simulink library "ddm"  (R2021b)
settings: Solver=VariableStepAuto  StartTime=0.0  StopTime=10.0  RelTol=1e-3
undefined symbols (not defined in the file or in its folder): ADDM_FrTMTqDev_X_Nm, ADDM_RrTMTqDev_X_Nm, ENUM_ADASACCSTA_ERROR, ENUM_ADASACCSTA_OFF, ENUM_ADASACCSTA_STANDBY, ENUM_ALLOWMOV_ALLOWREADY, ENUM_APS, ENUM_BRKSTA_ERROR, ENUM_BRKSTA_OFF, ENUM_BRKSTA_ON, ENUM_BRKSW_INVALID, ENUM_BRKSW_OFF, ENUM_BRKSW_ON, ENUM_CHGPREACTERRSTA_OBCPRE, ENUM_DCDCFAULTSTA_ANYFAULTLV1, ENUM_DCDCFAULTSTA_ANYFAULTLV2, ENUM_DRIVETRAIN_AWD, ENUM_DRIVETRAIN_FWD, ENUM_DRIVETRAIN_RWD, ENUM_EDUDRTSTA_NORMAL, ENUM_EPBSTA_APPLIED, ENUM_EPBSTA_RELEASED, ENUM_GEARACTUALPOSN_INVALID, ENUM_GEARACTUALPOSN_P, ENUM_HVBATTREADYPRE_READY, ENUM_MCUWARN_LV0, ENUM_MCUWARN_LV1, ENUM_MCUWARN_LV2, ENUM_MCUWARN_LV3, ENUM_MCUWARN_NOERROR, ENUM_OBCFAULTSTA_ANYFAULT, ENUM_PAS_R2F2, ENUM_PDFAULT_BATTPDFAIL, ENUM_PDFAULT_DCDCDISABLE, ENUM_PDFAULT_MCUDISABLE, ENUM_PDFAULT_MCUDISCHRG, ENUM_POWERSTA_OFF, ENUM_POWERSTA_ON, ENUM_POWERSTA_READY, ENUM_POWERSTA_STANDBY, ENUM_PRESSINDI_LOW, ENUM_PUFAULT_BATTUPFAIL, ENUM_PUFAULT_DCDCENABLEFAIL, ENUM_PUFAULT_PRECHRGCHKFAIL, ENUM_PUFAULT_SAFETYCHKFAIL, ENUM_PUSTATE_COMPLETED, ENUM_PWRSTASW_OFF, ENUM_PWRSTASW_OFFA, ENUM_PWRSTASW_OFFCHVCHRG, ENUM_PWRSTASW_OFFCLVCHRG, ENUM_PWRSTASW_ON, ENUM_PWRSTASW_ONHVCHRG, ENUM_PWRSTASW_READY, ENUM_PWRSTASW_STANDBY, ENUM_SHIFTCOMMAND_P, ENUM_SHIFTERERRSTA_PBUTTONFAILURE, ENUM_VEHMALFUNLV_2ND, ENUM_VEHMALFUNLV_3RD, ENUM_VEHMALFUNLV_4TH, ENUM_VEHMALFUNLV_NORMAL ... (+459)
libraries: hcu_lib x515, simulink x3
(part 1 of 25)
settings Model: VariantFading=off  Creator=13615  LastModifiedBy=FVT23033
settings SolverCC: AlgebraicLoopSolver=TrustRegion
settings DataIOCC: SaveFormat=Array  SignalLoggingSaveFormat=ModelDataLogs  ReturnWorkspaceOutputs=off
settings OptimizationCC: BlockReduction=off  BooleanDataType=off
settings DebuggingCC: SaveWithParameterizedLinksMsg=none  UnderspecifiedInitializationDetection=Classic  MergeDetectMultiDrivingBlocksExec=none  SignalResolutionControl=TryResolveAllWithWarning  SFMachineParentedDataDiag=warning  ArithmeticOperatorsInVariantConditions=warning
settings HardwareCC: TargetUnknown=on
settings ModelReferenceCC: PropagateSignalLabelsOutOfModel=off
settings SFSimCC: SimUseLocalCustomCode=off  CustomCodeUndefinedFunction=UseInterfaceOnly
settings RTWCC: RTWUseLocalCustomCode=off
settings ConfigComp: CovMetricSettings=dw  CovSaveCumulativeToWorkspaceVar=on  CovSaveSingleToWorkspaceVar=on

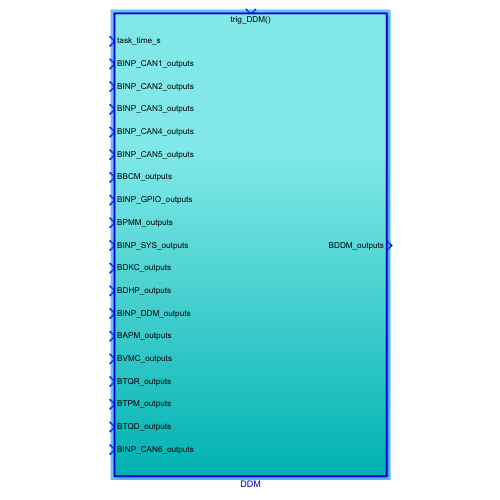
[thumbnail: Simulink's stored preview of the top-level diagram]
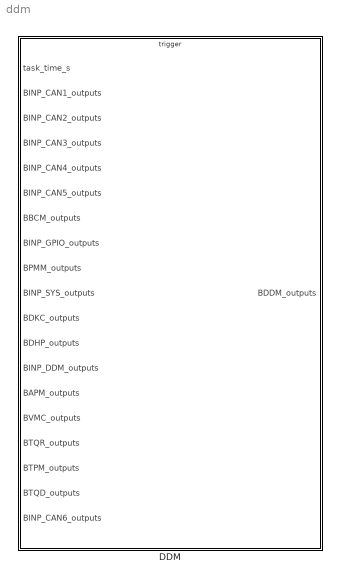
== system ddm ==
  DDM : Subsystem
      settings: RTWSystemCode=Nonreusable function  RTWFcnNameOpts=Use subsystem name  RTWFileNameOpts=Use subsystem name

== system ddm/DDM ==
  task_time_s : Inport
  BINP_CAN1_outputs : Inport  Port=2  OutDataTypeStr=Bus: BINP_CAN1_outputs
  BINP_CAN2_outputs : Inport  Port=3  OutDataTypeStr=Bus: BINP_CAN2_outputs
  BINP_CAN3_outputs : Inport  Port=4  OutDataTypeStr=Bus: BINP_CAN3_outputs
  BINP_CAN4_outputs : Inport  Port=5  OutDataTypeStr=Bus: BINP_CAN4_outputs
  BINP_CAN5_outputs : Inport  Port=6  OutDataTypeStr=Bus: BINP_CAN5_outputs
  BBCM_outputs : Inport  Port=7  OutDataTypeStr=Bus: BBCM_outputs
  BINP_GPIO_outputs : Inport  Port=8  OutDataTypeStr=Bus: BINP_GPIO_outputs
  BPMM_outputs : Inport  Port=9  OutDataTypeStr=Bus: BPMM_outputs
  BINP_SYS_outputs : Inport  Port=10  OutDataTypeStr=Bus: BINP_SYS_outputs
  BDKC_outputs : Inport  Port=11  OutDataTypeStr=Bus: BDKC_outputs
  BDHP_outputs : Inport  Port=12  OutDataTypeStr=Bus: BDHP_outputs
  BINP_DDM_outputs : Inport  Port=13  OutDataTypeStr=Bus: BINP_DDM_outputs
  BAPM_outputs : Inport  Port=14  OutDataTypeStr=Bus: BAPM_outputs
  BVMC_outputs : Inport  Port=15  OutDataTypeStr=Bus: BVMC_outputs
  BTQR_outputs : Inport  Port=16  OutDataTypeStr=Bus: BTQR_outputs
  BTPM_outputs : Inport  Port=17  OutDataTypeStr=Bus: BTPM_outputs
  BTQD_outputs : Inport  Port=18  OutDataTypeStr=Bus: BTQD_outputs
  BINP_CAN6_outputs : Inport  Port=19  OutDataTypeStr=Bus: BINP_CAN6_outputs
  trig_DDM : TriggerPort  TriggerType=function-call  VariantControl=(inherit)
  Bus Creator : BusCreator  Inputs=173  OutDataTypeStr=Bus: BDDM_outputs  NonVirtualBus=on
  Bus Selector : BusSelector  OutputSignals=VINP_CANMsgValidABM1_flg,VINP_BrkPedalPosSta_flg,VINP_BrkPedalPos_pct,VINP_BrkSwSta_flg,VINP_CANMsgValidESC1_flg,VINP_CANMsgValidESC5_flg,VINP_VehSpeed_kph,VINP_ESC1RCErr_flg,VINP_ESC1CSErr_flg,VINP_ESC5RCErr_flg,VINP_ESC5CSErr_flg,VINP_ABM1RCErr_flg,VINP_ABM1CSErr_flg,VINP_EPBSta_enum,VINP_EPBErrSta_enum,VINP_EBDFailed_flg,VINP_HDDFailed_flg,VINP_ABSFailed_flg,VINP_TCSFailed_flg,VINP_ESCFailed_flg,VINP_HBBFailed_flg,VINP_PBAFailed_flg,VINP_HSAFailed_flg,VINP_AVHFailed_flg,VINP_MCPressureV_flg,VINP_BrkSwV_flg,VINP_BrkPedalPosSta_flg,VINP_LongAccelV_flg,VINP_LatAccelV_flg,VINP_YawRateV_flg,VINP_RFPulseCountV_flg,VINP_RRPulseCountV_flg,VINP_LFPulseCountV_flg,VINP_LRPulseCountV_flg,VINP_LRRawWhlSpeedV_flg,VINP_RRRawWhlSpeedV_flg,VINP_LFRawWhlSpeedV_flg,VINP_RFRawWhlSpeedV_flg,VINP_CANMsgValidEPS1_flg,VINP_SASV_flg,VINP_CANMsgValidEPB1_flg,VINP_EPB1RCErr_flg,VINP_EPB1CSErr_flg,VINP_EPS1RCErr_flg,VINP_EPS1CSErr_flg
  Bus Selector1 : BusSelector  OutputSignals=VDHP_EAPCRBAD_flg,VDHP_EAPS1BAD_flg,VDHP_EAPS2BAD_flg,VDHP_EAPS12RangeSta_enum
  Bus Selector10 : BusSelector  OutputSignals=VDKC_DKCAuthSta_enum
  Bus Selector11 : BusSelector  OutputSignals=VVMC_ADASActive_flg,VVMC_APSActive_flg
  Bus Selector12 : BusSelector  OutputSignals=VTQR_FrTMTqReq_Nm,VTQR_RrTMTqReq_Nm
  Bus Selector13 : BusSelector  OutputSignals=VTPM_LFBatWarn_flg,VTPM_RFBatWarn_flg,VTPM_LRBatWarn_flg,VTPM_RRBatWarn_flg,VTPM_LFPressIndi_enum,VTPM_RFPressIndi_enum,VTPM_LRPressIndi_enum,VTPM_RRPressIndi_enum,VTPM_LFWheelTmpIndi_flg,VTPM_RFWheelTmpIndi_flg,VTPM_LRWheelTmpIndi_flg,VTPM_RRWheelTmpIndi_flg,VTPM_LFSensorFail_flg,VTPM_RFSensorFail_flg,VTPM_LRSensorFail_flg,VTPM_RRSensorFail_flg
  Bus Selector14 : BusSelector  OutputSignals=VTQD_ActParkRequest_flg,VTQD_SpdCtrlMode_enum,VTQD_GearActualPosn_enum,VTQD_ExternalTqAllow_flg,VTQD_ExtDoorAllow_flg
  Bus Selector15 : BusSelector  OutputSignals=VINP_CANMsgValidFCM1_flg,VINP_FCM1LifeCount_enum,VINP_FCM1Checksum_enum,VINP_ADASACCSta_enum,VINP_ACCRequiredAccel_mps2
  Bus Selector2 : BusSelector  OutputSignals=VINP_CANMsgValidBMS1_flg,VINP_CANMsgValidBMS6_flg,VINP_CANMsgValidCCU1_flg,VINP_CANMsgValidCCU2_flg,VINP_BMSWarn1_flg,VINP_BMSWarn2_flg,VINP_BMSWarn3_flg,VINP_BMSWarn4_flg,VINP_BMSWarn5_flg,VINP_BMSWarn6_flg,VINP_BMSWarn7_flg,VINP_BMSWarn8_flg,VINP_DCDCFaultSta_enum,VINP_OBCFaultSta_enum,VINP_MCUWarnFNidec_enum,VINP_MCUWarnRNidec_enum,VINP_LVBattDet12V_V,VINP_BMSREADY_flg,VINP_HVBattReady4Pre_enum,VINP_HVBContactorSta_flg,VINP_DCDCReady4Pre_flg,VINP_DCDCEnaSta_flg,VINP_CANMsgValidMCUNF1_flg,VINP_CANMsgValidMCUNR1_flg,VINP_CANMsgValidShifter1_flg,VINP_FrEDUDrtStaNidec_flg,VINP_FrEDURealTMTqNidec_Nm,VINP_RrEDUDrtStaNidec_flg,VINP_RrEDURealTMTqNidec_Nm,VINP_BMS6RCErr_flg,VINP_BMS6CSErr_flg,VINP_BMS1RCErr_flg,VINP_BMS1CSErr_flg,VINP_CCU1RCErr_flg,VINP_CCU1CSErr_flg,VINP_CCU2RCErr_flg,VINP_CCU2CSErr_flg,VINP_MCUNF1RCErr_flg,VINP_MCUNF1CSErr_flg,VINP_MCUNR1RCErr_flg,VINP_MCUNR1CSErr_flg,VINP_Shifter1RCErr_flg,VINP_Shifter1CSErr_flg,VINP_HVBattSOC_pct,VINP_ShifterHandleCmd_enum,VINP_ShifterFailsta_enum,VINP_CANMsgValidBMS5_flg
  Bus Selector3 : BusSelector  OutputSignals=VINP_ClearDTCcmd_flg
  Bus Selector4 : BusSelector  OutputSignals=VBCM_DiagHCrash_flg,VBCM_DiagFLTS_flg,VBCM_DiagFRTS_flg,VBCM_DiagRLTS_flg,VBCM_DiagRRTS_flg
  Bus Selector5 : BusSelector  OutputSignals=VAPM_USSStaFCL_flg,VAPM_USSStaFML_flg,VAPM_USSStaFMR_flg,VAPM_USSStaFCR_flg,VAPM_USSStaRCL_flg,VAPM_USSStaRML_flg,VAPM_USSStaRMR_flg,VAPM_USSStaRCR_flg,VAPM_USSStaFLL_flg,VAPM_USSStaFLR_flg,VAPM_USSStaRLL_flg,VAPM_USSStaRLR_flg,VAPM_SNSRLayout_enum
  Bus Selector6 : BusSelector  OutputSignals=VINP_DrStdAErrSta_flg,VINP_ZoneDrMalfunLevel_enum,VINP_CANMsgValidZONEDRVCU_flg,VINP_CANMsgValidZONEFRVCU_flg,VINP_CANMsgValidDKC1_flg,VINP_CANMsgValidDKC2_flg
  Bus Selector7 : BusSelector  OutputSignals=VINP_BrakeSWGPIO_flg,VINP_BrakeLampSW_flg,VINP_SeatSW_flg,VINP_DrDoorSW_flg,VINP_PsDoorSW_flg,VINP_RLDoorSW_flg,VINP_RRDoorSW_flg,VINP_HoodSW_flg,VINP_TailgateSW_flg,VINP_AccelPedal1Vol_V,VINP_AccelPedal2Vol_V
  Bus Selector8 : BusSelector  OutputSignals=VPMM_PowerSta_enum,VPMM_SysPowerMode_enum,VPMM_PowerUpFault_enum,VPMM_PowerDownFault_enum,VPMM_DrivetrainSelect_enum,VPMM_SafetyChkHLv_flg,VPMM_SafetyChkMLv_flg,VPMM_HVChrgPreActionErrSta_enum,VPMM_MCUReady_flg,VPMM_MCUReady4Pre_flg,VPMM_PowerUpState_enum,VPMM_MCUDCBusMaxVolt_V
  Bus Selector9 : BusSelector  OutputSignals=VINP_AllowMovThd_OTA_enum,VINP_Pedal1Ref5V_V,VINP_Pedal2Ref5V_V,VINP_AuxBattVolmV_mV,VINP_CAN1BusOff_flg,VINP_CAN3BusOff_flg,VINP_CAN4BusOff_flg,VINP_CAN6BusOff_flg
  Constant5 : Constant  Value=ZoneFrMalfunLevel_enum
  DDM : Subsystem
  Ground : Ground
  Terminator : Terminator
  Terminator2 : Terminator
  BDDM_outputs : Outport  OutDataTypeStr=Bus: BDDM_outputs
  wires:
  Bus Selector2/45 -> DDM/91(VINP_ShifterHandleCmd_enum)  "<VINP_ShifterHandleCmd_enum>"
  Bus Selector/14 -> DDM/15(VINP_EPBSta_enum)  "<VINP_EPBSta_enum>"
  Bus Selector14/1 -> DDM/177(VTQD_ActParkRequest_flg)  "<VTQD_ActParkRequest_flg>"
  BTQD_outputs/1 -> Bus Selector14/1
  Bus Selector9/4 -> DDM/121(VINP_AuxBattVolmV_mV)  "<VINP_AuxBattVolmV_mV>"
  Bus Selector2/44 -> DDM/90(VINP_HVBattSOC_pct)  "<VINP_HVBattSOC_pct>"
  Bus Selector9/3 -> DDM/120(VINP_Pedal2Ref5V_V)  "<VINP_Pedal2Ref5V_V>"
  Bus Selector9/2 -> DDM/119(VINP_Pedal1Ref5V_V)  "<VINP_Pedal1Ref5V_V>"
  Bus Selector13/16 -> DDM/176(VTPM_RRSensorFail_flg)  "<VTPM_RRSensorFail_flg>"
  Bus Selector13/15 -> DDM/175(VTPM_LRSensorFail_flg)  "<VTPM_LRSensorFail_flg>"
  Bus Selector13/14 -> DDM/174(VTPM_RFSensorFail_flg)  "<VTPM_RFSensorFail_flg>"
  Bus Selector13/13 -> DDM/173(VTPM_LFSensorFail_flg)  "<VTPM_LFSensorFail_flg>"
  Bus Selector5/13 -> DDM/149(VAPM_SNSRLayout_enum)  "<VAPM_SNSRLayout_enum>"
  Bus Selector13/12 -> DDM/172(VTPM_RRWheelTmpIndi_flg)  "<VTPM_RRWheelTmpIndi_flg>"
  Bus Selector13/11 -> DDM/171(VTPM_LRWheelTmpIndi_flg)  "<VTPM_LRWheelTmpIndi_flg>"
  Bus Selector13/10 -> DDM/170(VTPM_RFWheelTmpIndi_flg)  "<VTPM_RFWheelTmpIndi_flg>"
  Bus Selector13/9 -> DDM/169(VTPM_LFWheelTmpIndi_flg)  "<VTPM_LFWheelTmpIndi_flg>"
  Bus Selector13/8 -> DDM/168(VTPM_RRPressIndi_enum)  "<VTPM_RRPressIndi_enum>"
  Bus Selector13/7 -> DDM/167(VTPM_LRPressIndi_enum)  "<VTPM_LRPressIndi_enum>"
  Bus Selector13/6 -> DDM/166(VTPM_RFPressIndi_enum)  "<VTPM_RFPressIndi_enum>"
  Bus Selector13/5 -> DDM/165(VTPM_LFPressIndi_enum)  "<VTPM_LFPressIndi_enum>"
  Bus Selector/13 -> DDM/14(VDDM_C1ABM1CSChk_flg)  "<VINP_ABM1CSErr_flg>"
  Bus Selector/12 -> DDM/13(VDDM_C1ABM1RCChk_flg)  "<VINP_ABM1RCErr_flg>"
  Bus Selector/11 -> DDM/12(VDDM_ESC5CSErr_flg)  "<VINP_ESC5CSErr_flg>"
  Bus Selector/10 -> DDM/11(VDDM_ESC5RCErr_flg)  "<VINP_ESC5RCErr_flg>"
  Bus Selector/9 -> DDM/10(VDDM_ESC1CSErr_flg)  "<VINP_ESC1CSErr_flg>"
  Bus Selector/8 -> DDM/9(VDDM_ESC1RCErr_flg)  "<VINP_ESC1RCErr_flg>"
  Bus Selector2/43 -> DDM/89(VDDM_Shifter1CSErr_flg)  "<VINP_Shifter1CSErr_flg>"
  Bus Selector2/42 -> DDM/88(VDDM_Shifter1RCErr_flg)  "<VINP_Shifter1RCErr_flg>"
  Bus Selector2/41 -> DDM/87(VDDM_MCUNR1CSErr_flg)  "<VINP_MCUNR1CSErr_flg>"
  Bus Selector2/40 -> DDM/86(VDDM_MCUNR1RCErr_flg)  "<VINP_MCUNR1RCErr_flg>"
  Bus Selector2/39 -> DDM/85(VDDM_MCUNF1CSErr_flg)  "<VINP_MCUNF1CSErr_flg>"
  Bus Selector2/38 -> DDM/84(VDDM_MCUNF1RCErr_flg)  "<VINP_MCUNF1RCErr_flg>"
  Bus Selector2/37 -> DDM/83(VDDM_C3CCU2CSChk_flg)  "<VINP_CCU2CSErr_flg>"
  Bus Selector2/36 -> DDM/82(VDDM_C3CCU2RCChk_flg)  "<VINP_CCU2RCErr_flg>"
  Bus Selector2/35 -> DDM/81(VDDM_C3CCU1CSChk_flg)  "<VINP_CCU1CSErr_flg>"
  Bus Selector2/34 -> DDM/80(VDDM_C3CCU1RCChk_flg)  "<VINP_CCU1RCErr_flg>"
  Bus Selector2/33 -> DDM/79(VDDM_C3BMS1CSChk_flg)  "<VINP_BMS1CSErr_flg>"
  Bus Selector2/32 -> DDM/78(VDDM_C3BMS1RCChk_flg)  "<VINP_BMS1RCErr_flg>"
  Bus Selector2/31 -> DDM/77(VDDM_C3BMS6CSChk_flg)  "<VINP_BMS6CSErr_flg>"
  Bus Selector2/30 -> DDM/76(VDDM_C3BMS6RCChk_flg)  "<VINP_BMS6RCErr_flg>"
  Bus Selector13/4 -> DDM/164(VTPM_RRBatwarn_flg)  "<VTPM_RRBatWarn_flg>"
  Bus Selector13/3 -> DDM/163(VTPM_LRBatwarn_flg)  "<VTPM_LRBatWarn_flg>"
  Bus Selector13/2 -> DDM/162(VTPM_RFBatwarn_flg)  "<VTPM_RFBatWarn_flg>"
  Bus Selector13/1 -> DDM/161(VTPM_LFBatwarn_flg)  "<VTPM_LFBatWarn_flg>"
  BTPM_outputs/1 -> Bus Selector13/1
  Bus Selector12/2 -> DDM/160(VTQR_RrTMTqReq_Nm)  "<VTQR_RrTMTqReq_Nm>"
  Bus Selector12/1 -> DDM/159(VTQR_FrTMTqReq_Nm)  "<VTQR_FrTMTqReq_Nm>"
  BTQR_outputs/1 -> Bus Selector12/1
  Bus Selector2/29 -> DDM/75(VINP_RrEDURealTMTqNidec_Nm)  "<VINP_RrEDURealTMTqNidec_Nm>"
  Bus Selector2/28 -> DDM/74(VINP_RrEDUDrtStaNidec_flg)  "<VINP_RrEDUDrtStaNidec_flg>"
  Bus Selector2/27 -> DDM/73(VINP_FrEDURealTMTqNidec_Nm)  "<VINP_FrEDURealTMTqNidec_Nm>"
  Bus Selector2/26 -> DDM/72(VINP_FrEDUDrtStaNidec_flg)  "<VINP_FrEDUDrtStaNidec_flg>"
  Bus Selector/7 -> DDM/8(VINP_VehSpeed_kph)  "<VINP_VehSpeed_kph>"
  Bus Selector11/1 -> DDM/157(VVMC_ADASActive_flg)  "<VVMC_ADASActive_flg>"
  BVMC_outputs/1 -> Bus Selector11/1
  Bus Selector5/12 -> DDM/148(VAPM_USSStaRLR_flg)  "<VAPM_USSStaRLR_flg>"
  Bus Selector5/11 -> DDM/147(VAPM_USSStaRLL_flg)  "<VAPM_USSStaRLL_flg>"
  Bus Selector5/10 -> DDM/146(VAPM_USSStaFLR_flg)  "<VAPM_USSStaFLR_flg>"
  Bus Selector5/9 -> DDM/145(VAPM_USSStaFLL_flg)  "<VAPM_USSStaFLL_flg>"
  Bus Selector5/8 -> DDM/144(VAPM_USSStaRCR_flg)  "<VAPM_USSStaRCR_flg>"
  Bus Selector5/7 -> DDM/143(VAPM_USSStaRMR_flg)  "<VAPM_USSStaRMR_flg>"
  Bus Selector5/6 -> DDM/142(VAPM_USSStaRML_flg)  "<VAPM_USSStaRML_flg>"
  Bus Selector5/5 -> DDM/141(VAPM_USSStaRCL_flg)  "<VAPM_USSStaRCL_flg>"
  Bus Selector5/4 -> DDM/140(VAPM_USSStaFCR_flg)  "<VAPM_USSStaFCR_flg>"
  Bus Selector5/3 -> DDM/139(VAPM_USSStaFMR_flg)  "<VAPM_USSStaFMR_flg>"
  Bus Selector5/1 -> DDM/137(VAPM_USSStaFCL_flg)  "<VAPM_USSStaFCL_flg>"
  Bus Selector5/2 -> DDM/138(VAPM_USSStaFML_flg)  "<VAPM_USSStaFML_flg>"
  BAPM_outputs/1 -> Bus Selector5/1
  Bus Selector8/11 -> DDM/104(VPMM_PowerUpState_enum)  "<VPMM_PowerUpState_enum>"
  Bus Selector3/1 -> DDM/127(DTC_clear_request)  "<VINP_ClearDTCcmd_flg>"
  Bus Selector2/25 -> DDM/71(VINP_CANMsgValidShifter1_flg)  "<VINP_CANMsgValidShifter1_flg>"
  Bus Selector2/24 -> DDM/70(VINP_CANMsgValidMCUNR1_flg)  "<VINP_CANMsgValidMCUNR1_flg>"
  Bus Selector2/23 -> DDM/69(VINP_CANMsgValidMCUNF1_flg)  "<VINP_CANMsgValidMCUNF1_flg>"
  Bus Selector/6 -> DDM/7(VINP_CANMsgValidESC5_flg)  "<VINP_CANMsgValidESC5_flg>"
  Bus Selector/5 -> DDM/6(VINP_CANMsgValidESC1_flg)  "<VINP_CANMsgValidESC1_flg>"
  Bus Selector4/5 -> DDM/136(VBCM_DiagRRTS_flg)  "<VBCM_DiagRRTS_flg>"
  Bus Selector4/4 -> DDM/135(VBCM_DiagRLTS_flg)  "<VBCM_DiagRLTS_flg>"
  Bus Selector4/3 -> DDM/134(VBCM_DiagFRTS_flg)  "<VBCM_DiagFRTS_flg>"
  Bus Selector4/2 -> DDM/133(VBCM_DiagFLTS_flg)  "<VBCM_DiagFLTS_flg>"
  Bus Selector4/1 -> DDM/132(VBCM_DiagHCrash_flg)  "<VBCM_DiagHCrash_flg>"
  BINP_DDM_outputs/1 -> Bus Selector3/1
  Bus Selector8/10 -> DDM/103(VPMM_MCUReady4Pre_flg)  "<VPMM_MCUReady4Pre_flg>"
  Bus Selector8/9 -> DDM/102(VPMM_MCUReady_flg)  "<VPMM_MCUReady_flg>"
  Bus Selector8/8 -> DDM/101(VPMM_HVChrgPreActionErrSta_enum)  "<VPMM_HVChrgPreActionErrSta_enum>"
  Bus Selector8/7 -> DDM/100(VPMM_SafetyChkMLv_flg)  "<VPMM_SafetyChkMLv_flg>"
  Bus Selector8/6 -> DDM/99(VPMM_SafetyChkHLv_flg)  "<VPMM_SafetyChkHLv_flg>"
  Bus Selector1/1 -> DDM/128(VDHP_EAPCRBAD_flg)  "<VDHP_EAPCRBAD_flg>"
  BDHP_outputs/1 -> Bus Selector1/1
  Bus Selector7/11 -> DDM/116(VINP_AccelPedal2Vol_V)  "<VINP_AccelPedal2Vol_V>"
  Bus Selector7/10 -> DDM/115(VINP_AccelPedal1Vol_V)  "<VINP_AccelPedal1Vol_V>"
  DDM/39(VDDM_LVSupHiDTC_raw32) -> Bus Creator/39
  DDM/38(VDDM_LVSupLoDTC_raw32) -> Bus Creator/38
  DDM/37(VDDM_IniLVLoDTC_raw32) -> Bus Creator/37
  DDM/36(VDDM_OBC4PreDTC_raw32) -> Bus Creator/36
  DDM/35(VDDM_MCUActDTC_raw32) -> Bus Creator/35
  DDM/34(VDDM_HVRlyOpDTC_raw32) -> Bus Creator/34
  DDM/33(VDDM_DCDCDisDTC_raw32) -> Bus Creator/33
  DDM/32(VDDM_MCUDisDTC_raw32) -> Bus Creator/32
  DDM/31(VDDM_MidLvSaChkDTC_raw32) -> Bus Creator/31
  DDM/30(VDDM_HiLvSaChkDTC_raw32) -> Bus Creator/30
  DDM/29(VDDM_DCDCEnaDTC_raw32) -> Bus Creator/29
  DDM/28(VDDM_BMSRdyDTC_raw32) -> Bus Creator/28
  DDM/27(VDDM_HVRlyCloDTC_raw32) -> Bus Creator/27
  DDM/26(VDDM_DCDC4PreDTC_raw32) -> Bus Creator/26
  DDM/25(VDDM_MCU4PreDTC_raw32) -> Bus Creator/25
  DDM/24(VDDM_HVB4PreDTC_raw32) -> Bus Creator/24
  DDM/23(VDDM_ONtoRdyDTC_raw32) -> Bus Creator/23
  DDM/22(VDDM_KeyAuthDTC_raw32) -> Bus Creator/22
  DDM/21(VDDM_BrkSWNoBacDTC_raw32) -> Bus Creator/21
  DDM/20(VDDM_BrkSWErrDTC_raw32) -> Bus Creator/20
  DDM/19(VDDM_Lv4ErrDTC_raw32) -> Bus Creator/19
  DDM/18(VDDM_Lv3ErrDTC_raw32) -> Bus Creator/18
  DDM/17(VDDM_Lv2ErrDTC_raw32) -> Bus Creator/17
  DDM/1(VDDM_C3BMS6RCDTC_raw32) -> Bus Creator/1
  DDM/16(VDDM_Lv1ErrDTC_raw32) -> Bus Creator/16
  DDM/2(VDDM_C3BMS6CSDTC_raw32) -> Bus Creator/2
  DDM/15(VDDM_C1ABM1LCDTC_raw32) -> Bus Creator/15
  DDM/3(VDDM_C3BMS6LCDTC_raw32) -> Bus Creator/3
  DDM/14(VDDM_C1ABM1CSDTC_raw32) -> Bus Creator/14
  DDM/4(VDDM_C3BMS1RCDTC_raw32) -> Bus Creator/4
  DDM/13(VDDM_C1ABM1RCDTC_raw32) -> Bus Creator/13
  DDM/5(VDDM_C3BMS1CSDTC_raw32) -> Bus Creator/5
  DDM/12(VDDM_C3CCU2LCDTC_raw32) -> Bus Creator/12
  DDM/6(VDDM_C3BMS1LCDTC_raw32) -> Bus Creator/6
  DDM/11(VDDM_C3CCU2CSDTC_raw32) -> Bus Creator/11
  DDM/7(VDDM_C3CCU1RCDTC_raw32) -> Bus Creator/7
  DDM/10(VDDM_C3CCU2RCDTC_raw32) -> Bus Creator/10
  DDM/8(VDDM_C3CCU1CSDTC_raw32) -> Bus Creator/8
  DDM/9(VDDM_C3CCU1LCDTC_raw32) -> Bus Creator/9
  BBCM_outputs/1 -> Bus Selector4/1
  BINP_CAN5_outputs/1 -> Terminator2/1
  BINP_CAN4_outputs/1 -> Bus Selector6/1
  BINP_CAN2_outputs/1 -> Terminator/1
  Bus Selector7/3 -> DDM/108(VINP_DrStSW)  "<VINP_SeatSW_flg>"
  Bus Selector7/4 -> DDM/109(VINP_FLAJARSW)  "<VINP_DrDoorSW_flg>"
  Bus Selector7/5 -> DDM/110(VINP_FRAJARSW)  "<VINP_PsDoorSW_flg>"
  Bus Selector7/6 -> DDM/111(VINP_RLAJARSW)  "<VINP_RLDoorSW_flg>"
  Bus Selector7/7 -> DDM/112(VINP_RRAJARSW)  "<VINP_RRDoorSW_flg>"
  Bus Selector7/8 -> DDM/113(VINP_HoodSW)  "<VINP_HoodSW_flg>"
  Bus Selector7/9 -> DDM/114(VINP_TailgaSW)  "<VINP_TailgateSW_flg>"
  Bus Selector/4 -> DDM/5(VINP_BrkSWSta_flg)  "<VINP_BrkSwSta_flg>"
  Bus Selector2/22 -> DDM/68(VINP_DCDCEnabled_flg)  "<VINP_DCDCEnaSta_flg>"
  Bus Selector10/1 -> DDM/117(VDKC_DKCAuthSta_enum)  "<VDKC_DKCAuthSta_enum>"
  BDKC_outputs/1 -> Bus Selector10/1
  Bus Selector9/1 -> DDM/118(VINP_AllowMovThd_OTA_enum)  "<VINP_AllowMovThd_OTA_enum>"
  BINP_SYS_outputs/1 -> Bus Selector9/1
  Bus Selector7/2 -> DDM/107(VINP_BrakeLampSW_flg)  "<VINP_BrakeLampSW_flg>"
  Bus Selector7/1 -> DDM/106(VINP_BrakeSWGPIO_flg)  "<VINP_BrakeSWGPIO_flg>"
  Bus Selector8/5 -> DDM/98(VPMM_DrivetrainSelect_enum)  "<VPMM_DrivetrainSelect_enum>"
  Bus Selector8/4 -> DDM/97(VPMM_PowerDownFault_enum)  "<VPMM_PowerDownFault_enum>"
  Bus Selector8/3 -> DDM/96(VPMM_PowerUpFault_enum)  "<VPMM_PowerUpFault_enum>"
  Bus Selector8/2 -> DDM/95(VPMM_PwrStaSW_enum)  "<VPMM_SysPowerMode_enum>"
  Bus Selector8/1 -> DDM/94(VPMM_PowerSta_enum)  "<VPMM_PowerSta_enum>"
  Bus Selector2/21 -> DDM/67(VINP_DCDCReady4Pre_flg)  "<VINP_DCDCReady4Pre_flg>"
  Bus Selector2/20 -> DDM/66(VINP_HVBContactorSta_flg)  "<VINP_HVBContactorSta_flg>"
  Bus Selector2/19 -> DDM/65(VINP_HVBattReady4Pre_enum)  "<VINP_HVBattReady4Pre_enum>"
  Bus Selector2/18 -> DDM/64(VINP_BMSREADY_flg)  "<VINP_BMSREADY_flg>"
  Bus Selector2/17 -> DDM/63(VINP_LVBattDet12V_V)  "<VINP_LVBattDet12V_V>"
  Bus Selector2/16 -> DDM/62(VINP_MCUWarnRNidec_enum)  "<VINP_MCUWarnRNidec_enum>"
  Bus Selector2/15 -> DDM/61(VINP_MCUWarnFNidec_enum)  "<VINP_MCUWarnFNidec_enum>"
  Bus Selector2/14 -> DDM/60(VINP_OBCFaultSta_enum)  "<VINP_OBCFaultSta_enum>"
  Bus Selector2/13 -> DDM/59(VINP_DCDCFaultSta_enum)  "<VINP_DCDCFaultSta_enum>"
  Bus Selector2/12 -> DDM/58(VINP_BMSWarn8_flg)  "<VINP_BMSWarn8_flg>"
  Bus Selector2/11 -> DDM/57(VINP_BMSWarn7_flg)  "<VINP_BMSWarn7_flg>"
  Bus Selector2/10 -> DDM/56(VINP_BMSWarn6_flg)  "<VINP_BMSWarn6_flg>"
  Bus Selector2/9 -> DDM/55(VINP_BMSWarn5_flg)  "<VINP_BMSWarn5_flg>"
  Bus Selector2/8 -> DDM/54(VINP_BMSWarn4_flg)  "<VINP_BMSWarn4_flg>"
  Bus Selector2/7 -> DDM/53(VINP_BMSWarn3_flg)  "<VINP_BMSWarn3_flg>"
  Bus Selector2/6 -> DDM/52(VINP_BMSWarn2_flg)  "<VINP_BMSWarn2_flg>"
  Bus Selector2/1 -> DDM/47(VINP_CANMsgValidBMS1_flg)  "<VINP_CANMsgValidBMS1_flg>"
  Bus Selector2/5 -> DDM/51(VINP_BMSWarn1_flg)  "<VINP_BMSWarn1_flg>"
  Bus Selector2/2 -> DDM/48(VINP_CANMsgValidBMS6_flg)  "<VINP_CANMsgValidBMS6_flg>"
  Bus Selector2/4 -> DDM/50(VINP_CANMsgValidCCU2_flg)  "<VINP_CANMsgValidCCU2_flg>"
  Bus Selector2/3 -> DDM/49(VINP_CANMsgValidCCU1_flg)  "<VINP_CANMsgValidCCU1_flg>"
  Bus Selector/3 -> DDM/4(VINP_BrkPedalPos_pct)  "<VINP_BrkPedalPos_pct>"
  Bus Selector/2 -> DDM/3(VINP_BrkPedalPosSta_enum)  "<VINP_BrkPedalPosSta_flg>"
  Bus Selector/1 -> DDM/2(VINP_CANMsgValidABM1_flg)  "<VINP_CANMsgValidABM1_flg>"
  BPMM_outputs/1 -> Bus Selector8/1
  Bus Creator/1 -> BDDM_outputs/1  "BDDM_outputs"
  task_time_s/1 -> DDM/1(task_time_s)
  BINP_GPIO_outputs/1 -> Bus Selector7/1
  BINP_CAN3_outputs/1 -> Bus Selector2/1
  BINP_CAN1_outputs/1 -> Bus Selector/1
  Bus Selector6/1 -> DDM/150(VINP_DrStdAErrSta_enum)  "<VINP_DrStdAErrSta_flg>"
  Bus Selector6/2 -> DDM/151(VINP_ZoneDrMalfunLevel_enum)  "<VINP_ZoneDrMalfunLevel_enum>"
  Bus Selector15/1 -> DDM/182(VINP_CANMsgValidFCM1_flg)  "<VINP_CANMsgValidFCM1_flg>"
  Bus Selector14/2 -> DDM/178(VINP_ZoneSpdCtrlMode_enum)  "<VTQD_SpdCtrlMode_enum>"
  Bus Selector2/46 -> DDM/92(VINP_ShifterFailsta_enum)  "<VINP_ShifterFailsta_enum>"
  Constant5/1 -> DDM/156(ZoneFrMalfunLevel_enum)
  Bus Selector8/12 -> DDM/105(VPMM_MCUDCBusMaxVolt_V)  "<VPMM_MCUDCBusMaxVolt_V>"
  Bus Selector14/3 -> DDM/179(VTQD_GearActualPosn_enum)  "<VTQD_GearActualPosn_enum>"
  Bus Selector/15 -> DDM/16(VINP_EPBErrSta_enum)  "<VINP_EPBErrSta_enum>"
  Bus Selector/41 -> DDM/42(VINP_CANMsgValidEPB1_flg)  "<VINP_CANMsgValidEPB1_flg>"
  Bus Selector1/2 -> DDM/129(VDHP_EAPS1BAD_flg)  "<VDHP_EAPS1BAD_flg>"
  Bus Selector1/3 -> DDM/130(VDHP_EAPS2BAD_flg)  "<VDHP_EAPS2BAD_flg>"
  BINP_CAN6_outputs/1 -> Bus Selector15/1
  Bus Selector15/2 -> DDM/183(VDDM_FCM1RCErr_flg)  "<VINP_FCM1LifeCount_enum>"
  Bus Selector15/3 -> DDM/184(VDDM_FCM1CSErr_flg)  "<VINP_FCM1Checksum_enum>"
  Bus Selector15/4 -> DDM/185(VINP_ADASACCSta_enum)  "<VINP_ADASACCSta_enum>"
  Bus Selector15/5 -> DDM/186(VINP_ACCRequireAccel_mps2)  "<VINP_ACCRequiredAccel_mps2>"
  Bus Selector14/4 -> DDM/180(VTQD_ExternalTqAllow_flg)  "<VTQD_ExternalTqAllow_flg>"
  Bus Selector14/5 -> DDM/181(VTQD_ExtDoorAllow_flg)  "<VTQD_ExtDoorAllow_flg>"
  Bus Selector/38 -> DDM/39(VINP_RFRawWhlSpeedV_flg)  "<VINP_RFRawWhlSpeedV_flg>"
  Bus Selector/37 -> DDM/38(VINP_LFRawWhlSpeedV_flg)  "<VINP_LFRawWhlSpeedV_flg>"
  Bus Selector/36 -> DDM/37(VINP_RRRawWhlSpeedV_flg)  "<VINP_RRRawWhlSpeedV_flg>"
  Bus Selector/35 -> DDM/36(VINP_LRRawWhlSpeedV_flg)  "<VINP_LRRawWhlSpeedV_flg>"
  Bus Selector/34 -> DDM/35(VINP_LRPulseCountV_flg)  "<VINP_LRPulseCountV_flg>"
  Bus Selector/33 -> DDM/34(VINP_LFPulseCountV_flg)  "<VINP_LFPulseCountV_flg>"
  Bus Selector/32 -> DDM/33(VINP_RRPulseCountV_flg)  "<VINP_RRPulseCountV_flg>"
  Bus Selector/31 -> DDM/32(VINP_RFPulseCountV_flg)  "<VINP_RFPulseCountV_flg>"
  Bus Selector/30 -> DDM/31(VINP_YawRateV_flg)  "<VINP_YawRateV_flg>"
  Bus Selector/29 -> DDM/30(VINP_LatAccelV_flg)  "<VINP_LatAccelV_flg>"
  Bus Selector/28 -> DDM/29(VINP_LongAccelV_flg)  "<VINP_LongAccelV_flg>"
  Bus Selector/27 -> DDM/28(VINP_BrkPedalPosSta_flg)  "<VINP_BrkPedalPosSta_flg>"
  Bus Selector/26 -> DDM/27(VINP_BrkSwV_flg)  "<VINP_BrkSwV_flg>"
  Bus Selector/25 -> DDM/26(VINP_MCPressureV_flg)  "<VINP_MCPressureV_flg>"
  Bus Selector/24 -> DDM/25(VINP_AVHFailed_flg)  "<VINP_AVHFailed_flg>"
  Bus Selector/23 -> DDM/24(VINP_HSAFailed_flg)  "<VINP_HSAFailed_flg>"
  Bus Selector/22 -> DDM/23(VINP_PBAFailed_flg)  "<VINP_PBAFailed_flg>"
  Bus Selector/21 -> DDM/22(VINP_HBBFailed_flg)  "<VINP_HBBFailed_flg>"
  Bus Selector/20 -> DDM/21(VINP_ESCFailed_flg)  "<VINP_ESCFailed_flg>"
  Bus Selector/19 -> DDM/20(VINP_TCSFailed_flg)  "<VINP_TCSFailed_flg>"
  Bus Selector/18 -> DDM/19(VINP_ABSFailed_flg)  "<VINP_ABSFailed_flg>"
  Bus Selector/17 -> DDM/18(VINP_HDDFailed_flg)  "<VINP_HDDFailed_flg>"
  Bus Selector/16 -> DDM/17(VINP_EBDFailed_flg)  "<VINP_EBDFailed_flg>"
  Bus Selector/39 -> DDM/40(VINP_CANMsgValidEPS1_flg)  "<VINP_CANMsgValidEPS1_flg>"
  Bus Selector/40 -> DDM/41(VINP_SASV_flg)  "<VINP_SASV_flg>"
  DDM/40(VDDM_LVInErrDTC_raw32) -> Bus Creator/40
  DDM/41(VDDM_DrStSWDTC_raw32) -> Bus Creator/41
  DDM/42(VDDM_FLDoorSWDTC_raw32) -> Bus Creator/42
  DDM/43(VDDM_RLDoorSWDTC_raw32) -> Bus Creator/43
  DDM/44(VDDM_FRDoorSWDTC_raw32) -> Bus Creator/44
  DDM/45(VDDM_RRDoorSWDTC_raw32) -> Bus Creator/45
  DDM/46(VDDM_HoodSWDTC_raw32) -> Bus Creator/46
  DDM/47(VDDM_TailgaSWDTC_raw32) -> Bus Creator/47
  DDM/48(VDDM_EDriveSysErrVCUErr_flg) -> Bus Creator/48
  DDM/49(VDDM_VehMalfunLevel_enum) -> Bus Creator/49
  DDM/50(VDDM_APS1SigOoRDTC_raw32) -> Bus Creator/50
  DDM/51(VDDM_APS2SigOoRDTC_raw32) -> Bus Creator/51
  DDM/52(VDDM_APSCorrErrDTC_raw32) -> Bus Creator/52
  DDM/53(VDDM_MCUF1NoComDTC_raw32) -> Bus Creator/53
  DDM/54(VDDM_MCUR1NoComDTC_raw32) -> Bus Creator/54
  DDM/55(VDDM_Shifter1NoComDTC_raw32) -> Bus Creator/55
  DDM/56(VDDM_ESC7NoComDTC_raw32) -> Bus Creator/56
  DDM/57(VDDM_ESC1NoComDTC_raw32) -> Bus Creator/57
  DDM/58(VDDM_ESC5NoComDTC_raw32) -> Bus Creator/58
  DDM/59(VDDM_EnterNewOperCyc_flg) -> Bus Creator/59
  DDM/60(VDDM_DiagHCrashDTC_raw32) -> Bus Creator/60
  DDM/61(VDDM_DiagFLTSDTC_raw32) -> Bus Creator/61
  DDM/62(VDDM_DiagFRTSDTC_raw32) -> Bus Creator/62
  DDM/63(VDDM_DiagRLTSDTC_raw32) -> Bus Creator/63
  DDM/64(VDDM_DiagRRTSDTC_raw32) -> Bus Creator/64
  DDM/65(VDDM_FCLUSSDTC_raw32) -> Bus Creator/65
  DDM/66(VDDM_FMLUSSDTC_raw32) -> Bus Creator/66
  DDM/67(VDDM_FMRUSSDTC_raw32) -> Bus Creator/67
  DDM/68(VDDM_FCRUSSDTC_raw32) -> Bus Creator/68
  DDM/69(VDDM_RCLUSSDTC_raw32) -> Bus Creator/69
  DDM/70(VDDM_RMLUSSDTC_raw32) -> Bus Creator/70
  DDM/71(VDDM_RMRUSSDTC_raw32) -> Bus Creator/71
  DDM/72(VDDM_RCRUSSDTC_raw32) -> Bus Creator/72
  DDM/73(VDDM_FLLUSSDTC_raw32) -> Bus Creator/73
  DDM/74(VDDM_FLRUSSDTC_raw32) -> Bus Creator/74
  DDM/75(VDDM_RLLUSSDTC_raw32) -> Bus Creator/75
  DDM/76(VDDM_RLRUSSDTC_raw32) -> Bus Creator/76
  DDM/77(VDDM_FCM2NoComDTC_raw32) -> Bus Creator/77
  DDM/78(VDDM_FCM2RCErrDTC_raw32) -> Bus Creator/78
  DDM/79(VDDM_FCM2CSErrDTC_raw32) -> Bus Creator/79
  DDM/81(VDDM_FCM3RCErrDTC_raw32) -> Bus Creator/81
  DDM/80(VDDM_FCM3NoComDTC_raw32) -> Bus Creator/80
  DDM/82(VDDM_FCM3CSErrDTC_raw32) -> Bus Creator/82
  DDM/83(VDDM_FCM4NoComDTC_raw32) -> Bus Creator/83
  DDM/84(VDDM_FCM4CSErrDTC_raw32) -> Bus Creator/84
  DDM/85(VDDM_FCM5NoComDTC_raw32) -> Bus Creator/85
  DDM/86(VDDM_FCM5CSErrDTC_raw32) -> Bus Creator/86
  DDM/87(VDDM_ZoneSCPNoComDTC_raw32) -> Bus Creator/87
  DDM/88(VDDM_BMSSigErrDetDTC_raw32) -> Bus Creator/88
  DDM/89(VDDM_FCMACCSigErrDetDTC_raw32) -> Bus Creator/89
  DDM/90(VDDM_FrMCUSigErrDetDTC_raw32) -> Bus Creator/90
  DDM/91(VDDM_RrMCUSigErrDetDTC_raw32) -> Bus Creator/91
  DDM/92(VDDM_CCUSigErrDetDTC_raw32) -> Bus Creator/92
  DDM/93(VDDM_ACCAccelCmdErrDetDTC_raw32) -> Bus Creator/93
  DDM/94(VDDM_ACCMalfuncDetDTC_raw32) -> Bus Creator/94
  DDM/95(VDDM_CCMalfuncDetDTC_raw32) -> Bus Creator/95
  DDM/96(VDDM_MSAMalfuncDetDTC_raw32) -> Bus Creator/96
  DDM/97(VDDM_ISAMalfuncDetDTC_raw32) -> Bus Creator/97
  DDM/98(VDDM_MCUF1RCErrDTC_raw32) -> Bus Creator/98
  DDM/99(VDDM_MCUR1RCErrDTC_raw32) -> Bus Creator/99
  DDM/100(VDDM_MCUF1CSErrDTC_raw32) -> Bus Creator/100
  DDM/101(VDDM_MCUR1CSErrDTC_raw32) -> Bus Creator/101
  DDM/102(VDDM_Shifter1RCErrDTC_raw32) -> Bus Creator/102
  DDM/103(VDDM_Shifter1CSErrDTC_raw32) -> Bus Creator/103
  DDM/104(VDDM_ESC7RCErrDTC_raw32) -> Bus Creator/104
  DDM/105(VDDM_ESC7CSErrDTC_raw32) -> Bus Creator/105
  DDM/106(VDDM_ESC1RCErrDTC_raw32) -> Bus Creator/106
  DDM/107(VDDM_ESC1CSErrDTC_raw32) -> Bus Creator/107
  DDM/108(VDDM_ESC5RCErrDTC_raw32) -> Bus Creator/108
  DDM/109(VDDM_ESC5C  SErrDTC_raw32) -> Bus Creator/109
  DDM/110(VDDM_FrMCUTqErrDTC_raw32) -> Bus Creator/110
  DDM/111(VDDM_RrMCUTqErrDTC_raw32) -> Bus Creator/111
  DDM/112(VDDM_LFBatwarnDTC_raw32) -> Bus Creator/112
  DDM/113(VDDM_RFBatwarnDTC_raw32) -> Bus Creator/113
  DDM/114(VDDM_LRBatwarnDTC_raw32) -> Bus Creator/114
  DDM/115(VDDM_RRBatwarnDTC_raw32) -> Bus Creator/115
  DDM/116(VDDM_LFPressIndiDTC_raw32) -> Bus Creator/116
  DDM/117(VDDM_RFPressIndiDTC_raw32) -> Bus Creator/117
  DDM/118(VDDM_LRPressIndiDTC_raw32) -> Bus Creator/118
  DDM/119(VDDM_RRPressIndiDTC_raw32) -> Bus Creator/119
  DDM/120(VDDM_LFWheelTmpHighDTC_raw32) -> Bus Creator/120
  DDM/121(VDDM_RFWheelTmpHighDTC_raw32) -> Bus Creator/121
  DDM/122(VDDM_LRWheelTmpHighDTC_raw32) -> Bus Creator/122
  DDM/123(VDDM_RRWheelTmpHighDTC_raw32) -> Bus Creator/123
  DDM/124(VDDM_LFSensorFailDTC_raw32) -> Bus Creator/124
  DDM/125(VDDM_RFSensorFailDTC_raw32) -> Bus Creator/125
  DDM/126(VDDM_LRSensorFailDTC_raw32) -> Bus Creator/126
  DDM/127(VDDM_RRSensorFailDTC_raw32) -> Bus Creator/127
  DDM/128(VDDM_C1EPAS2LCDTC_raw32) -> Bus Creator/128
  DDM/129(VDDM_5vAPS1PwrErrDTC_raw32) -> Bus Creator/129
  DDM/151(VDDM_EPSSigErrDTC_raw32) -> Bus Creator/151
  DDM/150(VDDM_EPS1CSErrDTC_raw32) -> Bus Creator/150
  DDM/149(VDDM_EPS1RCErrDTC_raw32) -> Bus Creator/149
  DDM/148(VDDM_EPS1NoComDTC_raw32) -> Bus Creator/148
  DDM/147(VDDM_ZoneFrSigErrDetDTC_raw32) -> Bus Creator/147
  DDM/146(VDDM_ZoneDrSigErrDetDTC_raw32) -> Bus Creator/146
  DDM/145(VDDM_FrVCUNoComDTC_raw32) -> Bus Creator/145
  DDM/144(VDDM_DrVCUNoComDTC_raw32) -> Bus Creator/144
  DDM/143(VDDM_ShifterSigErrDetDTC_raw32) -> Bus Creator/143
  DDM/142(VDDM_ESCSigErrDetDTC_raw32) -> Bus Creator/142
  DDM/141(VDDM_FCM1CSErrDTC_raw32) -> Bus Creator/141
  DDM/140(VDDM_FCM1RCErrDTC_raw32) -> Bus Creator/140
  DDM/139(VDDM_FCM1NoComDTC_raw32) -> Bus Creator/139
  DDM/138(VDDM_EPBSigErrDTC_raw32) -> Bus Creator/138
  DDM/136(VDDM_EPB1RCErrDTC_raw32) -> Bus Creator/136
  DDM/137(VDDM_EPB1CSErrDTC_raw32) -> Bus Creator/137
  DDM/135(VDDM_EPB1NoComDTC_raw32) -> Bus Creator/135
  DDM/134(VDDM_EDriveSysErr_VCUErrTmp_flg) -> Bus Creator/134
  DDM/133(VDDM_LimpHomeActTmp_flg) -> Bus Creator/133
  DDM/132(VDDM_EPBUnlockTODTC_raw32) -> Bus Creator/132
  DDM/131(VDDM_EPBLockTODTC_raw32) -> Bus Creator/131
  DDM/130(VDDM_5vAPS2PwrErrDTC_raw32) -> Bus Creator/130
  Bus Selector6/3 -> DDM/152(VINP_CANMsgValidZoneDrVCU_flg)  "<VINP_CANMsgValidZONEDRVCU_flg>"
  Bus Selector6/4 -> DDM/153(VINP_CANMsgValidZoneFrVCU_flg)  "<VINP_CANMsgValidZONEFRVCU_flg>"
  Bus Selector2/47 -> DDM/93(VINP_CANMsgValidBMS5_flg)  "<VINP_CANMsgValidBMS5_flg>"
  DDM/152(VDDM_DTCDetect_enum) -> Bus Creator/152
  DDM/153(VDDM_EngagePFail_flg) -> Bus Creator/153
  DDM/154(VDDM_DisengagePFail_flg) -> Bus Creator/154
  DDM/155(VDDM_VCURAPSErrLv2_flg) -> Bus Creator/155
  DDM/156(VDDM_VCURAPSErrLv3_flg) -> Bus Creator/156
  Bus Selector1/4 -> DDM/131(VDHP_EAPS12RangeSta_enum)  "<VDHP_EAPS12RangeSta_enum>"
  DDM/157(VDDM_EDriveSysErrShifterErr_flg) -> Bus Creator/157
  Bus Selector6/5 -> DDM/154(VINP_CANMsgValidDKC1_flg)  "<VINP_CANMsgValidDKC1_flg>"
  Bus Selector6/6 -> DDM/155(VINP_CANMsgValidDKC2_flg)  "<VINP_CANMsgValidDKC2_flg>"
  DDM/158(VDDM_PMMBattErr_flg) -> Bus Creator/158
  DDM/159(VDDM_LVSysErrPwrOutErr_flg) -> Bus Creator/159
  Bus Selector11/2 -> DDM/158(VVMC_APSActive_flg)  "<VVMC_APSActive_flg>"
  DDM/160(VDDM_HVRlyOpFail_flg) -> Bus Creator/160
  DDM/161(VDDM_MCUActDisFail_flg) -> Bus Creator/161
  DDM/162(VDDM_VCUBrkSWSta_enum) -> Bus Creator/162
  DDM/163(VDDM_VCUFLDoorSta_flg) -> Bus Creator/163
  DDM/164(VDDM_VCUFRDoorSta_flg) -> Bus Creator/164
  DDM/165(VDDM_VCURLDoorSta_flg) -> Bus Creator/165
  DDM/166(VDDM_VCURRDoorSta_flg) -> Bus Creator/166
  DDM/167(VDDM_SysAllowReadySta_flg) -> Bus Creator/167
  DDM/168(VDDM_VCUHoodSWSta_flg) -> Bus Creator/168
  DDM/169(VDDM_VCUTailgateSWSta_flg) -> Bus Creator/169
  Bus Selector/42 -> DDM/43(VDDM_EPB1RCErr_flg)  "<VINP_EPB1RCErr_flg>"
  Bus Selector/43 -> DDM/44(VDDM_EPB1CSErr_flg)  "<VINP_EPB1CSErr_flg>"
  Bus Selector/44 -> DDM/45(VDDM_EPSRCErr_flg)  "<VINP_EPS1RCErr_flg>"
  Bus Selector/45 -> DDM/46(VDDM_EPSCSErr_flg)  "<VINP_EPS1CSErr_flg>"
  Bus Selector9/5 -> DDM/122(VINP_CAN1BusOff_flg)  "<VINP_CAN1BusOff_flg>"
  Bus Selector9/6 -> DDM/123(VINP_CAN3BusOff_flg)  "<VINP_CAN3BusOff_flg>"
  Bus Selector9/7 -> DDM/124(VINP_CAN4BusOff_flg)  "<VINP_CAN4BusOff_flg>"
  DDM/170(VDDM_EPB1NoComCFS_flg) -> Bus Creator/170
  DDM/171(VDDM_EPB1RCErrCFS_flg) -> Bus Creator/171
  DDM/172(VDDM_EPB1CSErrCFS_flg) -> Bus Creator/172
  DDM/173(VDDM_EPBSigErrCFS_flg) -> Bus Creator/173
  Ground/1 -> DDM/126(No_CAN_BUS_OFF)
  Bus Selector9/8 -> DDM/125(VINP_CAN6BusOff_flg)  "<VINP_CAN6BusOff_flg>"
